simulink model "LQR_Controller"  (R2023b)
settings: Solver=VariableStepAuto  StartTime=0.0  StopTime=20  RelTol=1e-3
settings Model: Creator=patel  LastModifiedBy=patel

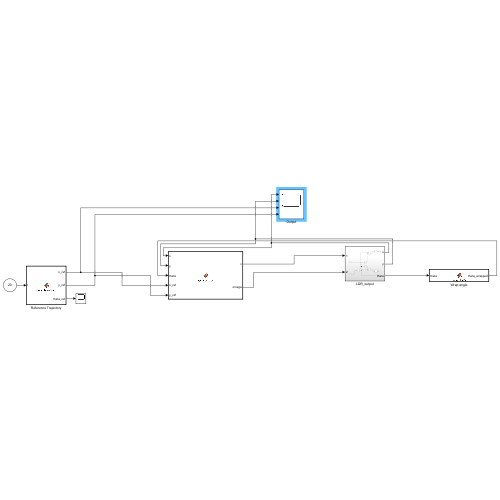
[thumbnail: Simulink's stored preview of the top-level diagram]
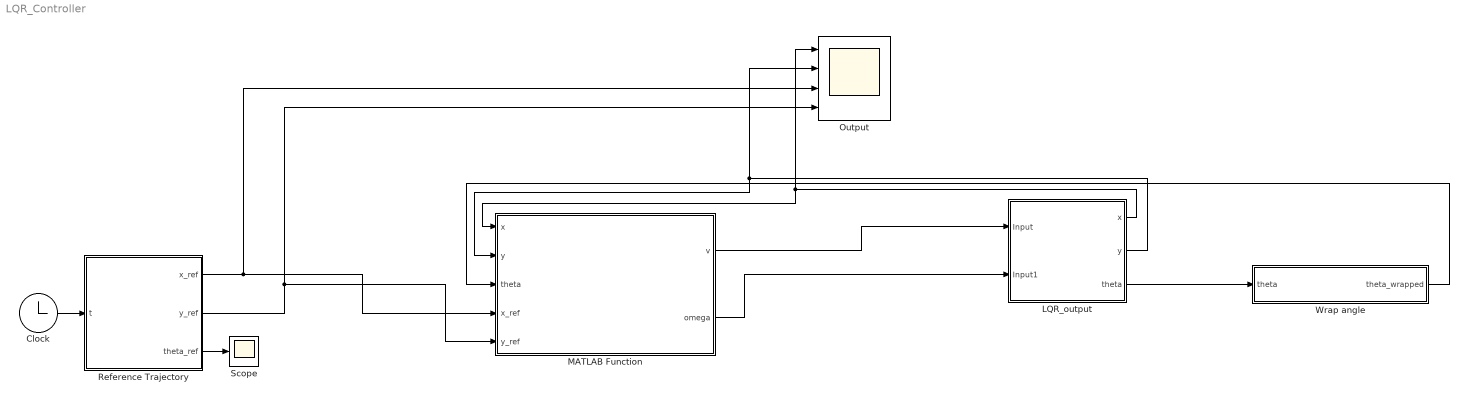
== system LQR_Controller ==
  Clock : Clock
      settings: Decimation=20
  LQR_output : Subsystem
  MATLAB Function : MATLAB Function  TreatAsAtomicUnit=on
  Output : Scope  NumInputPorts=4
  Reference Trajectory : MATLAB Function  TreatAsAtomicUnit=on
  Scope : Scope
  Wrap angle : MATLAB Function  TreatAsAtomicUnit=on
  wires:
  Wrap angle/1(theta_wrapped) -> MATLAB Function/3(theta)
  MATLAB Function/1(v) -> LQR_output/1(Input)
  Reference Trajectory/1(x_ref) -> Output/3, MATLAB Function/4(x_ref)
  LQR_output/2(y) -> MATLAB Function/2(y), Output/2
  Clock/1 -> Reference Trajectory/1(t)
  Reference Trajectory/3(theta_ref) -> Scope/1
  Reference Trajectory/2(y_ref) -> Output/4, MATLAB Function/5(y_ref)
  LQR_output/1(x) -> MATLAB Function/1(x), Output/1
  MATLAB Function/2(omega) -> LQR_output/2(Input1)
  LQR_output/3(theta) -> Wrap angle/1(theta)

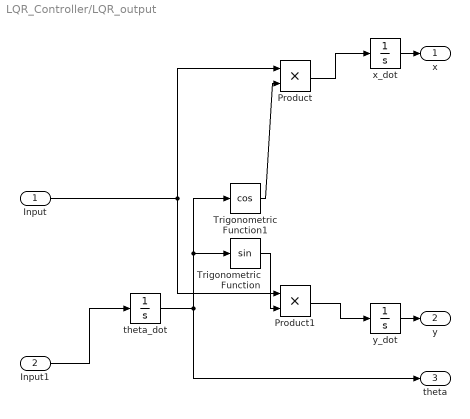
== system LQR_Controller/LQR_output ==
  Input : Inport
  Input1 : Inport  Port=2
  Product : Product
  Product1 : Product
  Trigonometric Function : Trigonometry
  Trigonometric Function1 : Trigonometry  Operator=cos
  theta_dot : Integrator
  x_dot : Integrator
  y_dot : Integrator
  x : Outport
  y : Outport  Port=2
  theta : Outport  Port=3
  wires:
  theta_dot/1 -> theta/1, Trigonometric Function1/1, Trigonometric Function/1
  Product/1 -> x_dot/1
  Input1/1 -> theta_dot/1
  Trigonometric Function1/1 -> Product/2
  Input/1 -> Product1/1, Product/1
  Trigonometric Function/1 -> Product1/2
  Product1/1 -> y_dot/1
  x_dot/1 -> x/1
  y_dot/1 -> y/1

== matlab function LQR_Controller/Reference Trajectory ==
  data: t input; x_ref output; y_ref output; theta_ref output
function [x_ref, y_ref, theta_ref] = trajectoryGen(t)
    radius = 5;
    omega_ref = 0.2;
    x_ref = radius * cos(omega_ref * t);
    y_ref = radius * sin(omega_ref * t);
    theta_ref = omega_ref * t + pi/2;
end

== matlab function LQR_Controller/Wrap angle ==
  data: theta input; theta_wrapped output
function theta_wrapped = wrapToPi(theta)
    theta_wrapped = mod(theta + pi, 2*pi) - pi;
end

== matlab function LQR_Controller/MATLAB Function ==
  data: x input; v output; y input; theta input; x_ref input; y_ref input; omega output
function [v, omega] = lqr_control(x, y, theta, x_ref, y_ref)
%#codegen
robotState = [x; y; theta];
targetPoint = [x_ref; y_ref];
[v, omega] = LQRController(robotState, targetPoint);

function [v, omega] = LQRController(robotState, targetPoint)
    % Inputs:
    %   robotState = [x; y; theta]
    %   targetPoint = [x_target; y_target]

    x = robotState(1);
    y = robotState(2);
    theta = robotState(3);

    x_target = targetPoint(1);
    y_target = targetPoint(2);

    % LQR Gain matrix (2x3)
    K = [1.5, 0.0, 0.0;
         0.0, 1.5, 2.0];

    % Global error
    dx = x_target - x;
    dy = y_target - y;
    error_global = [dx; dy];

    % Rotation matrix to robot frame
    c = cos(theta);
    s = sin(theta);
    R = [c, s; -s, c];
    error_robot = R * error_global;

    % Theta error
    angle_to_target = atan2(dy, dx);
    theta_error = atan2(sin(angle_to_target - theta), cos(angle_to_target - theta));

    % Form error state
    error_state = [error_robot; theta_error];

    % Control input via LQR gains
    v_r = K(1, :) * error_state;
    v_l = K(2, :) * error_state;

    % Convert to unicycle model control inputs
    v = (v_r + v_l) / 2;
    omega = (v_r - v_l) / 0.2;  % 0.2m wheel base

    % Saturation
    v = max(0.2, min(v, 5.0));
    omega = min(max(omega, -pi), pi);
end
end
